simulink model "EV_model"  (R2024b)
settings: Solver=VariableStepAuto  StartTime=0.0  StopTime=60.0  RelTol=1e-3
libraries: simulink x1, SignalEditorBlockLib x1
settings Model: Creator=Pavithra M  LastModifiedBy=Pavithra M

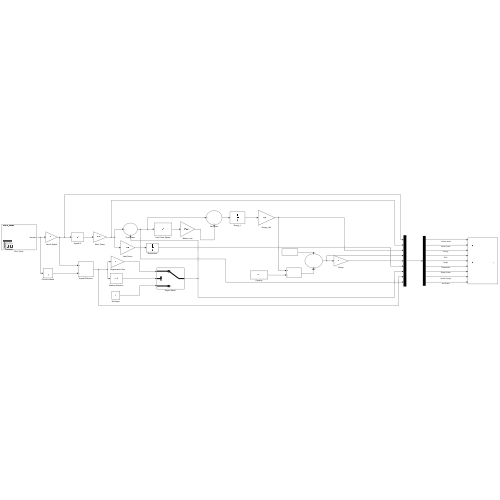
[thumbnail: Simulink's stored preview of the top-level diagram]
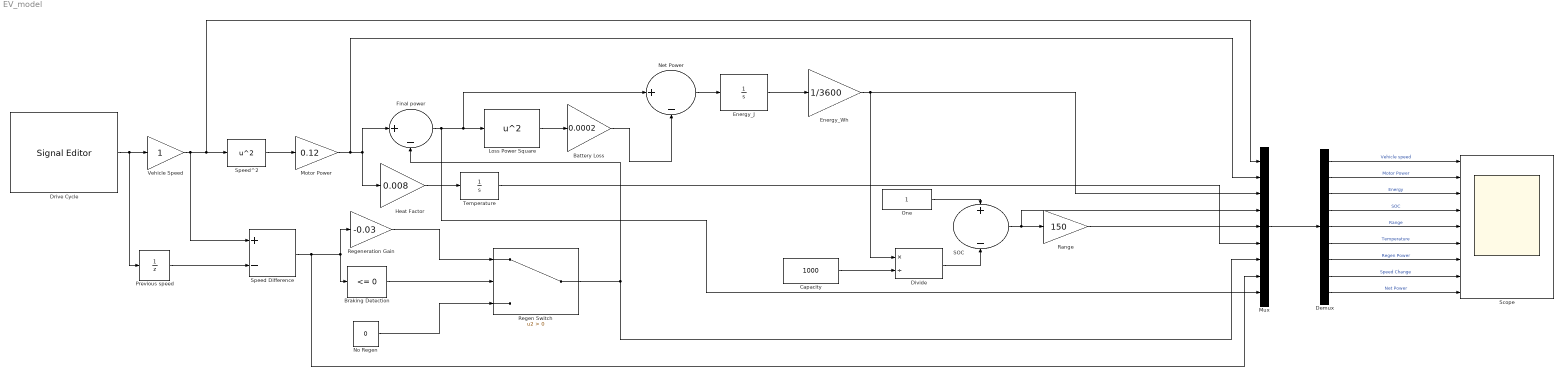
== system EV_model ==
  Battery Loss : Gain  Gain=0.0002
  Braking Detection : simulink/Logic and Bit Operations/Compare To Zero  relop=<=  OutDataTypeStr=boolean
  Capacity : Constant  Value=1000
  Demux : Demux  Outputs=9
  Divide : Product  Inputs=*/
  Drive Cycle : SignalEditorBlockLib/Signal Editor  FileName=C:\Users\Pavithra M\OneDrive\Desktop\drive_cycle.mat  ActiveScenario=Normal_Mode  ActiveSignal=Normal  IsBus=off  OutputBusObjectStr=Bus: BusObject  SampleTime=0  Interpolate=off  ZeroCross=off  OutputAfterFinalValue=Setting to zero  Unit=inherit  PreserveSignalName=on  ApplySigPropsToAllScenarios=on  ApplySigPropsToAllSignals=off
  Energy_J : Integrator
  Energy_Wh : Gain  Gain=1/3600
  Final power : Sum  Inputs=|+-
  Heat Factor : Gain  Gain=0.008
  Loss Power Square : Math  Operator=square
  Motor Power : Gain  Gain=0.12
  Mux : Mux  Inputs=9
  Net Power : Sum  Inputs=|+-
  No Regen : Constant  Value=0
  One : Constant
  Previous speed : UnitDelay  SampleTime=-1  HasFrameUpgradeWarning=on
  Range : Gain  Gain=150
  Regen Switch : Switch  Criteria=u2 > Threshold  SaturateOnIntegerOverflow=off  InputSameDT=off
  Regeneration Gain : Gain  Gain=-0.03
  SOC : Sum  Inputs=+-
  Scope : Scope  NumInputPorts=9
  Speed Difference : Sum  Inputs=+-
  Speed^2 : Math  Operator=square
  Temperature : Integrator
  Vehicle Speed : Gain
  wires:
  One/1 -> SOC/1
  Divide/1 -> SOC/2
  Energy_J/1 -> Energy_Wh/1
  Drive Cycle/1 -> Vehicle Speed/1, Previous speed/1
  Capacity/1 -> Divide/2
  Range/1 -> Mux/5
  Speed^2/1 -> Motor Power/1
  SOC/1 -> Range/1, Mux/4
  Energy_Wh/1 -> Divide/1, Mux/3
  Heat Factor/1 -> Temperature/1
  Vehicle Speed/1 -> Speed^2/1, Mux/1, Speed Difference/1
  Mux/1 -> Demux/1
  Demux/1 -> Scope/1  "Vehicle speed"
  Demux/2 -> Scope/2  "Motor Power"
  Demux/3 -> Scope/3  "Energy"
  Demux/4 -> Scope/4  "SOC"
  Demux/5 -> Scope/5  "Range"
  Demux/6 -> Scope/6  "Temperature"
  Temperature/1 -> Mux/6
  Previous speed/1 -> Speed Difference/2
  Speed Difference/1 -> Mux/8, Regeneration Gain/1, Braking Detection/1
  No Regen/1 -> Regen Switch/3
  Regen Switch/1 -> Mux/7, Final power/2
  Braking Detection/1 -> Regen Switch/2
  Regeneration Gain/1 -> Regen Switch/1
  Demux/7 -> Scope/7  "Regen Power"
  Demux/8 -> Scope/8  "Speed Change"
  Demux/9 -> Scope/9  "Net Power"
  Loss Power Square/1 -> Battery Loss/1
  Net Power/1 -> Energy_J/1
  Battery Loss/1 -> Net Power/2
  Motor Power/1 -> Heat Factor/1, Final power/1, Mux/2
  Final power/1 -> Loss Power Square/1, Net Power/1, Mux/9
